simulink model "Movimiento_traslacional"  (R2024a)
settings: Solver=VariableStepAuto  StartTime=0.0  StopTime=10.0  RelTol=1e-3
InitFcn:
  | m1=290;
  | b1=1000;
  | m2=59;
  | k1=16182;
  | f=0;
  | k2=19000;

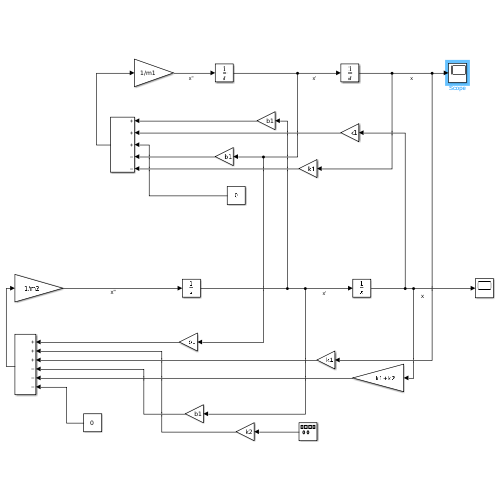
[thumbnail: Simulink's stored preview of the top-level diagram]
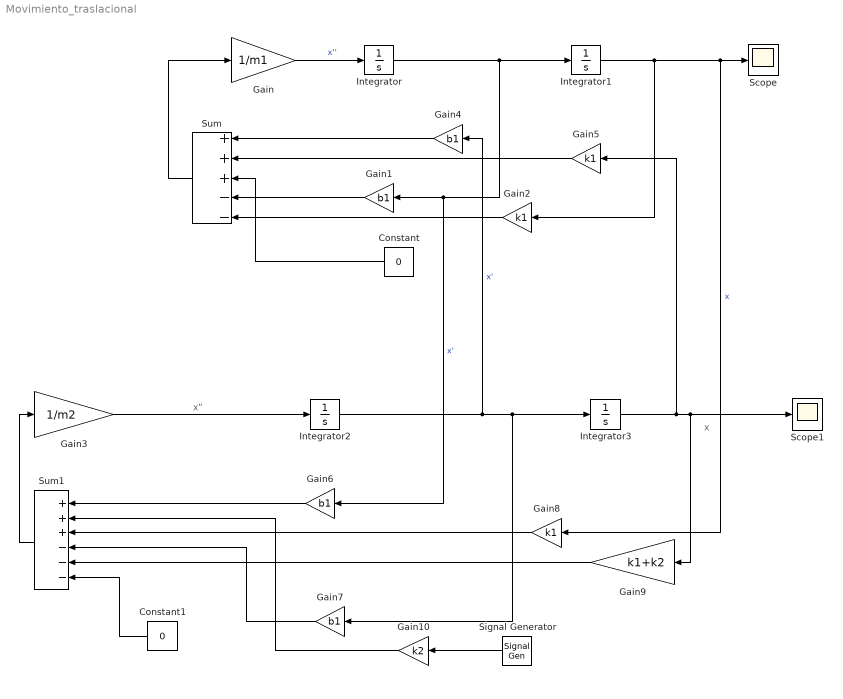
== system Movimiento_traslacional ==
  note: x
  note: x"
  Constant : Constant  Value=0
  Constant1 : Constant  Value=0
  Gain : Gain  Gain=1/m1
  Gain{1,4,6..7} (4 alike) : Gain  Gain=b1
  Gain10 : Gain  Gain=k2
  Gain2 : Gain  Gain=k1
  Gain3 : Gain  Gain=1/m2
  Gain5 : Gain  Gain=k1
  Gain8 : Gain  Gain=k1
  Gain9 : Gain  Gain=k1+k2
  Integrator{,1..3} (4 alike) : Integrator
  Scope : Scope
  Scope1 : Scope
  Signal Generator : SignalGenerator  Amplitude=0.05  Frequency=0.5*pi  Units=rad/sec
  Sum : Sum  Inputs=+++--
  Sum1 : Sum  Inputs=+++---
  wires:
  Integrator/1 -> Gain6/1, Gain1/1, Integrator1/1  "x'"
  Integrator1/1 -> Gain8/1, Scope/1, Gain2/1  "x"
  Gain/1 -> Integrator/1  "x''"
  Gain1/1 -> Sum/4
  Sum/1 -> Gain/1
  Constant/1 -> Sum/3
  Gain2/1 -> Sum/5
  Integrator2/1 -> Gain4/1, Gain7/1, Integrator3/1  "x'"
  Integrator3/1 -> Gain9/1, Scope1/1, Gain5/1
  Gain3/1 -> Integrator2/1
  Sum1/1 -> Gain3/1
  Constant1/1 -> Sum1/6
  Gain4/1 -> Sum/1
  Gain5/1 -> Sum/2
  Gain6/1 -> Sum1/1
  Gain7/1 -> Sum1/4
  Gain8/1 -> Sum1/3
  Gain9/1 -> Sum1/5
  Gain10/1 -> Sum1/2
  Signal Generator/1 -> Gain10/1
